simulink model "Multi_Robot_MPC_Adaptive"  (R2018a)
settings: Solver=VariableStepAuto  StartTime=0.0  StopTime=inf  FixedStep=sampleTime  RelTol=1e-3
PreLoadFcn:
  | % Simulation parameters
  | load exampleMap
  | sampleTime = 0.05;
  | 
  | % Robot parameters
  | wheelRadius = 0.025;
  | robotRadius = 0.35;
  | 
  | % Lidar parameters
  | sensorOffset = [0,0];
  | scanAngles = linspace(-pi/2,pi/2,9)';
  | maxRange = 5;
undefined symbols (not defined in the file): Ad, Bd, Beta, C1, C2, cBW, d, dw, Kb, Kg, Kt, L, La, magnitude, mc, R, Ra, Waypoint
libraries: mobileRoboticsLib x7, cstblocks x1, dspsrcs4 x1
settings Model: EnablePacing=on  Creator=scastro  LastModifiedBy=shravan

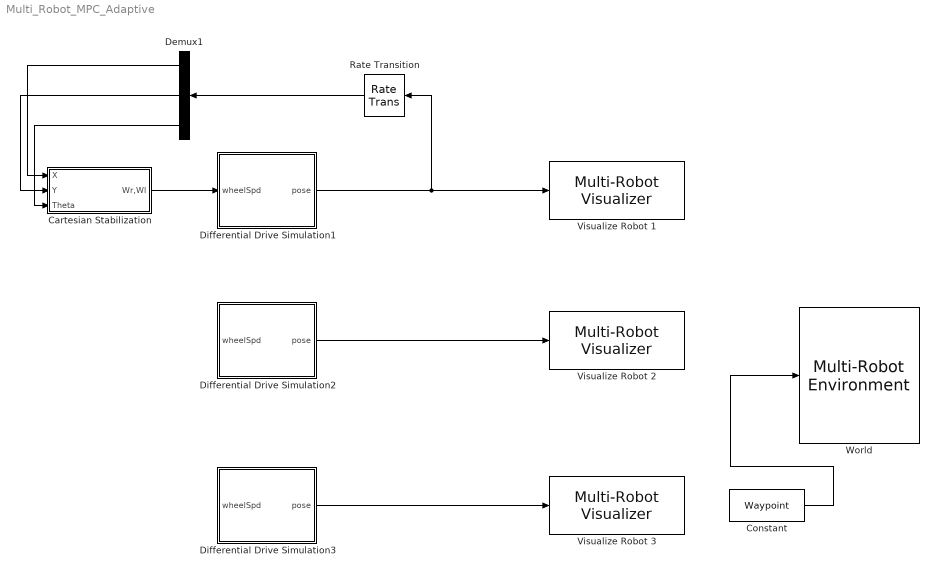
== system Multi_Robot_MPC_Adaptive ==
  Cartesian Stabilization : Subsystem
  Constant : Constant  Value=Waypoint  SampleTime=sampleTime
  Demux1 : Demux  Outputs=3
  Differential Drive Simulation1 : Subsystem  AncestorBlock=mobileRoboticsLib/Kinematic Models/Differential Drive/Differential Drive Simulation  OverrideUsingVariant=mode==2  mask(Differential Drive Simulation){wheelRadius=R, wheelBase=L, initX=C1, initY=C2, initAngle=0, Ts=0}
      mask prompts: wheelRadius "Wheel Radius [m]"; wheelBase "Wheelbase [m]"; initX "Initial X Position [m]"; initY "Initial Y Position [m]"; initAngle "Initial Angle [rad]"; Ts "Sample Time"
      mask help:
      | Simulates the kinematics of a differential drive vehicle from a specified initial pose.
      |
      | Input: Left and right wheel speeds [wL; wR], in rad/s
      |
      | Output: Pose [x; y; theta], in m, m, and rad
      |
      | Set the Sample Time parameter to 0 for continuous-time simulation, or a positive number for discrete-time simulation.
      mask Help: web('matlab:edit mrsDocDifferentialDrive')
      mask Callback Ts:
      | Ts = evalin('base',get_param(gcb,'Ts'));
      | blk = [gcb '/Generic Robot Simulation/Velocity Integrator'];
      | if Ts > 0
      |     set_param(blk,'OverrideUsingVariant','mode==2');
      | else
      |     set_param(blk,'OverrideUsingVariant','mode==1');
      | end
  Differential Drive Simulation2 : Subsystem  AncestorBlock=mobileRoboticsLib/Kinematic Models/Differential Drive/Differential Drive Simulation  OverrideUsingVariant=mode==2  mask(Differential Drive Simulation){wheelRadius=R, wheelBase=L, initX=C1, initY=C2+1, initAngle=0, Ts=0}
      mask prompts: wheelRadius "Wheel Radius [m]"; wheelBase "Wheelbase [m]"; initX "Initial X Position [m]"; initY "Initial Y Position [m]"; initAngle "Initial Angle [rad]"; Ts "Sample Time"
      mask help:
      | Simulates the kinematics of a differential drive vehicle from a specified initial pose.
      |
      | Input: Left and right wheel speeds [wL; wR], in rad/s
      |
      | Output: Pose [x; y; theta], in m, m, and rad
      |
      | Set the Sample Time parameter to 0 for continuous-time simulation, or a positive number for discrete-time simulation.
      mask Help: web('matlab:edit mrsDocDifferentialDrive')
      mask Callback Ts:
      | Ts = evalin('base',get_param(gcb,'Ts'));
      | blk = [gcb '/Generic Robot Simulation/Velocity Integrator'];
      | if Ts > 0
      |     set_param(blk,'OverrideUsingVariant','mode==2');
      | else
      |     set_param(blk,'OverrideUsingVariant','mode==1');
      | end
  Differential Drive Simulation3 : Subsystem  AncestorBlock=mobileRoboticsLib/Kinematic Models/Differential Drive/Differential Drive Simulation  OverrideUsingVariant=mode==2  mask(Differential Drive Simulation){wheelRadius=R, wheelBase=L, initX=C1, initY=C2-1, initAngle=0, Ts=0}
      mask prompts: wheelRadius "Wheel Radius [m]"; wheelBase "Wheelbase [m]"; initX "Initial X Position [m]"; initY "Initial Y Position [m]"; initAngle "Initial Angle [rad]"; Ts "Sample Time"
      mask help:
      | Simulates the kinematics of a differential drive vehicle from a specified initial pose.
      |
      | Input: Left and right wheel speeds [wL; wR], in rad/s
      |
      | Output: Pose [x; y; theta], in m, m, and rad
      |
      | Set the Sample Time parameter to 0 for continuous-time simulation, or a positive number for discrete-time simulation.
      mask Help: web('matlab:edit mrsDocDifferentialDrive')
      mask Callback Ts:
      | Ts = evalin('base',get_param(gcb,'Ts'));
      | blk = [gcb '/Generic Robot Simulation/Velocity Integrator'];
      | if Ts > 0
      |     set_param(blk,'OverrideUsingVariant','mode==2');
      | else
      |     set_param(blk,'OverrideUsingVariant','mode==1');
      | end
  Rate Transition : RateTransition  OutPortSampleTime=0.01
  Visualize Robot 1 : mobileRoboticsLib/Environments/Multi-Robot Visualizer  idx=1  radius=0.8  robotColor=[0 0 1]  showTraj=on  hasLidar=off  sensorOffset=[0 0]  scanAngles=[-pi/4,0,pi/4]  hasObjDetector=off  objDetectorOffset=[0;0]  objDetectorAngle=0  objDetectorFOV=pi/2  objDetectorMaxRange=5
      settings: SourceProductName=Mobile Robotics Simulation Toolbox
  Visualize Robot 2 : mobileRoboticsLib/Environments/Multi-Robot Visualizer  idx=2  radius=0.8  robotColor=[0 1 0]  showTraj=on  hasLidar=off  sensorOffset=[0 0]  scanAngles=[-pi/4,0,pi/4]  hasObjDetector=off  objDetectorOffset=[0;0]  objDetectorAngle=0  objDetectorFOV=pi/2  objDetectorMaxRange=5
      settings: SourceProductName=Mobile Robotics Simulation Toolbox
  Visualize Robot 3 : mobileRoboticsLib/Environments/Multi-Robot Visualizer  idx=3  radius=0.8  robotColor=[1 0 1]  showTraj=on  hasLidar=off  sensorOffset=[0 0]  scanAngles=[-pi/4,0,pi/4]  hasObjDetector=off  objDetectorOffset=[0;0]  objDetectorAngle=0  objDetectorFOV=pi/2  objDetectorMaxRange=5
      settings: SourceProductName=Mobile Robotics Simulation Toolbox
  World : mobileRoboticsLib/Environments/Multi-Robot Environment  numRobots=3  showWaypoints=on  showObjects=off  objectColors=[1 0 0;0 1 0;0 0 1]  objectMarkers='s'  showRobotIds=on  plotSensorLines=off
      settings: SourceProductName=Mobile Robotics Simulation Toolbox
  wires:
  Differential Drive Simulation1/1(pose) -> Rate Transition/1, Visualize Robot 1/1
  Cartesian Stabilization/1(Wr,Wl) -> Differential Drive Simulation1/1(wheelSpd)
  Rate Transition/1 -> Demux1/1
  Demux1/1 -> Cartesian Stabilization/1(X)
  Demux1/2 -> Cartesian Stabilization/2(Y)
  Demux1/3 -> Cartesian Stabilization/3(Theta)
  Differential Drive Simulation2/1(pose) -> Visualize Robot 2/1
  Differential Drive Simulation3/1(pose) -> Visualize Robot 3/1
  Constant/1 -> World/1

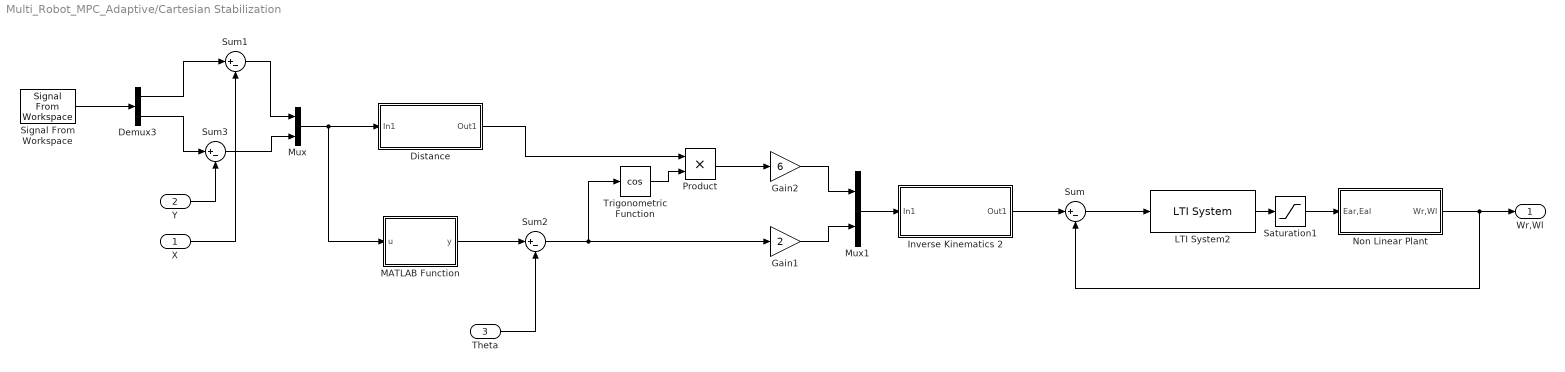
== system Multi_Robot_MPC_Adaptive/Cartesian Stabilization ==
  X : Inport
  Y : Inport  Port=2
  Theta : Inport  Port=3
  Demux3 : Demux  Outputs=2
  "Distance " : Subsystem
  Gain1 : Gain  Gain=2
  Gain2 : Gain  Gain=6
  Inverse Kinematics 2 : Subsystem
  LTI System2 : cstblocks/LTI System  sys=Controller  IC=[]
  MATLAB Function : MATLAB Function  TreatAsAtomicUnit=on
  Mux : Mux  Inputs=2
  Mux1 : Mux  Inputs=2
  "Non Linear Plant " : Subsystem
  Product : Product
  Saturation1 : Saturate  UpperLimit=30  LowerLimit=-30
  Signal From Workspace : dspsrcs4/Signal From Workspace  X=Cartesian  Ts=cBW  nsamps=1  OutputAfterFinalValue=Holding final value  ignoreOrWarnInputAndFrameLengths=off  OutputFrames=off
  Sum{,1..3} (4 alike) : Sum  Inputs=|+-
  Trigonometric Function : Trigonometry  Operator=cos
  Wr,Wl : Outport
  wires:
  "Distance "/1(Out1) -> Product/1
  Y/1 -> Sum3/2
  Demux3/1 -> Sum1/1
  Saturation1/1 -> "Non Linear Plant "/1(Ear,Eal)
  Gain2/1 -> Mux1/1
  Mux1/1 -> Inverse Kinematics 2/1(In1)
  Sum1/1 -> Mux/1
  Demux3/2 -> Sum3/1
  LTI System2/1 -> Saturation1/1
  Inverse Kinematics 2/1(Out1) -> Sum/1
  Signal From Workspace/1 -> Demux3/1
  Gain1/1 -> Mux1/2
  Sum3/1 -> Mux/2
  Theta/1 -> Sum2/2
  Sum/1 -> LTI System2/1
  "Non Linear Plant "/1(Wr,Wl) -> Wr,Wl/1, Sum/2
  Trigonometric Function/1 -> Product/2
  MATLAB Function/1(y) -> Sum2/1
  X/1 -> Sum1/2
  Product/1 -> Gain2/1
  Sum2/1 -> Gain1/1, Trigonometric Function/1
  Mux/1 -> MATLAB Function/1(u), "Distance "/1(In1)

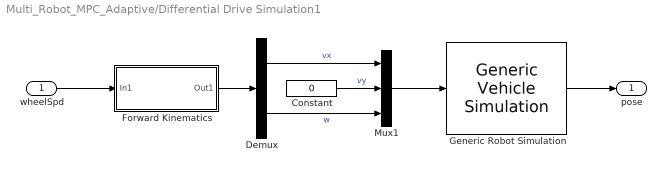
== system Multi_Robot_MPC_Adaptive/Differential Drive Simulation1 ==
  wheelSpd : Inport
  Constant : Constant  Value=0
  Demux : Demux  Outputs=2
  "Forward Kinematics " : Subsystem
  Generic Robot Simulation : mobileRoboticsLib/Utilities/Generic Vehicle Simulation  initX=initX  initY=initY  initAngle=initAngle  Ts=Ts
      link override Velocity Integrator: OverrideUsingVariant=mode==1
      settings: SourceProductName=Mobile Robotics Simulation Toolbox
  Mux1 : Mux  Inputs=3
  pose : Outport
  wires:
  Mux1/1 -> Generic Robot Simulation/1
  Demux/1 -> Mux1/1  "vx"
  Demux/2 -> Mux1/3  "w"
  Constant/1 -> Mux1/2  "vy"
  wheelSpd/1 -> "Forward Kinematics "/1(In1)
  "Forward Kinematics "/1(Out1) -> Demux/1
  Generic Robot Simulation/1 -> pose/1

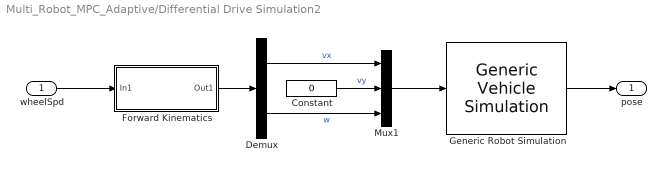
== system Multi_Robot_MPC_Adaptive/Differential Drive Simulation2 ==
  wheelSpd : Inport
  Constant : Constant  Value=0
  Demux : Demux  Outputs=2
  "Forward Kinematics " : Subsystem
  Generic Robot Simulation : mobileRoboticsLib/Utilities/Generic Vehicle Simulation  initX=initX  initY=initY  initAngle=initAngle  Ts=Ts
      link override Velocity Integrator: OverrideUsingVariant=mode==1
      settings: SourceProductName=Mobile Robotics Simulation Toolbox
  Mux1 : Mux  Inputs=3
  pose : Outport
  wires:
  Mux1/1 -> Generic Robot Simulation/1
  Demux/1 -> Mux1/1  "vx"
  Demux/2 -> Mux1/3  "w"
  Constant/1 -> Mux1/2  "vy"
  wheelSpd/1 -> "Forward Kinematics "/1(In1)
  "Forward Kinematics "/1(Out1) -> Demux/1
  Generic Robot Simulation/1 -> pose/1

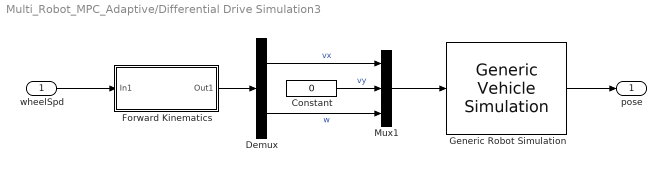
== system Multi_Robot_MPC_Adaptive/Differential Drive Simulation3 ==
  wheelSpd : Inport
  Constant : Constant  Value=0
  Demux : Demux  Outputs=2
  "Forward Kinematics " : Subsystem
  Generic Robot Simulation : mobileRoboticsLib/Utilities/Generic Vehicle Simulation  initX=initX  initY=initY  initAngle=initAngle  Ts=Ts
      link override Velocity Integrator: OverrideUsingVariant=mode==1
      settings: SourceProductName=Mobile Robotics Simulation Toolbox
  Mux1 : Mux  Inputs=3
  pose : Outport
  wires:
  Mux1/1 -> Generic Robot Simulation/1
  Demux/1 -> Mux1/1  "vx"
  Demux/2 -> Mux1/3  "w"
  Constant/1 -> Mux1/2  "vy"
  wheelSpd/1 -> "Forward Kinematics "/1(In1)
  "Forward Kinematics "/1(Out1) -> Demux/1
  Generic Robot Simulation/1 -> pose/1

== system Multi_Robot_MPC_Adaptive/Cartesian Stabilization/Distance  ==
  In1 : Inport
  Add2 : Sum
  Demux : Demux  Outputs=2
  Math Function : Math  Operator=magnitude^2  SaturateOnIntegerOverflow=on
  Math Function1 : Math  Operator=magnitude^2  SaturateOnIntegerOverflow=on
  Sqrt : Sqrt  SaturateOnIntegerOverflow=on
  Out1 : Outport
  wires:
  In1/1 -> Demux/1
  Demux/1 -> Math Function/1
  Demux/2 -> Math Function1/1
  Math Function/1 -> Add2/1
  Math Function1/1 -> Add2/2
  Add2/1 -> Sqrt/1
  Sqrt/1 -> Out1/1

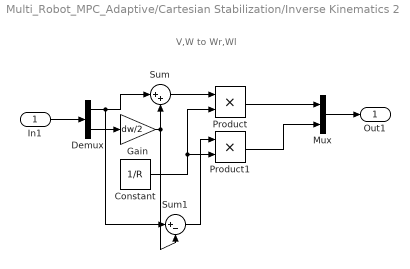
== system Multi_Robot_MPC_Adaptive/Cartesian Stabilization/Inverse Kinematics 2 ==
  note: V,W to Wr,Wl
  In1 : Inport
  Constant : Constant  Value=1/R
  Demux : Demux  Outputs=2
  Gain : Gain  Gain=dw/2
  Mux : Mux  Inputs=2
  Product : Product
  Product1 : Product
  Sum : Sum  Inputs=|++
  Sum1 : Sum  Inputs=|+-
  Out1 : Outport
  wires:
  Mux/1 -> Out1/1
  In1/1 -> Demux/1
  Demux/2 -> Gain/1
  Demux/1 -> Sum1/1, Sum/1
  Gain/1 -> Sum1/2, Sum/2
  Sum/1 -> Product/1
  Constant/1 -> Product1/2, Product/2
  Sum1/1 -> Product1/1
  Product/1 -> Mux/1
  Product1/1 -> Mux/2

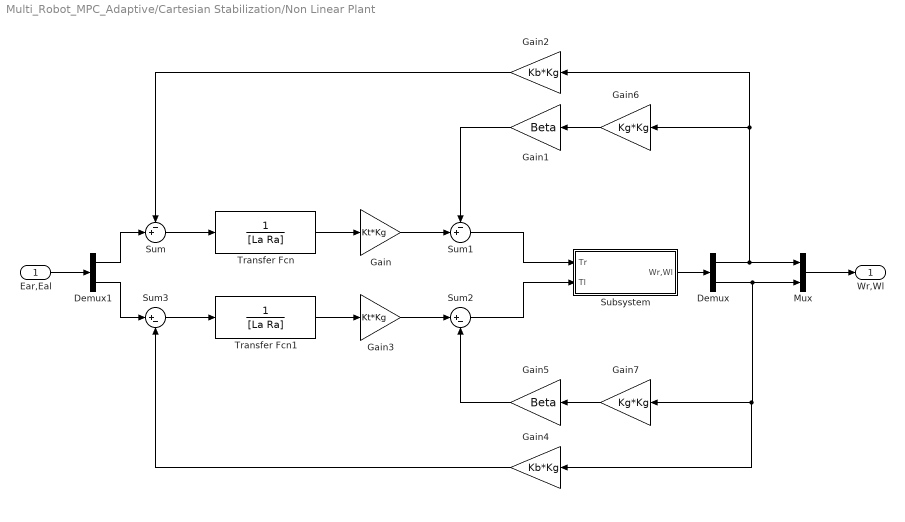
== system Multi_Robot_MPC_Adaptive/Cartesian Stabilization/Non Linear Plant  ==
  Ear,Eal : Inport
  Demux : Demux  Outputs=2
  Demux1 : Demux  Outputs=2
  Gain : Gain  Gain=Kt*Kg
  Gain1 : Gain  Gain=Beta
  Gain2 : Gain  Gain=Kb*Kg
  Gain3 : Gain  Gain=Kt*Kg
  Gain4 : Gain  Gain=Kb*Kg
  Gain5 : Gain  Gain=Beta
  Gain6 : Gain  Gain=Kg*Kg
  Gain7 : Gain  Gain=Kg*Kg
  Mux : Mux  Inputs=2
  Subsystem : Subsystem
  Sum : Sum  Inputs=-+|
  Sum1 : Sum  Inputs=-+|
  Sum2 : Sum  Inputs=|+-
  Sum3 : Sum  Inputs=|+-
  Transfer Fcn : TransferFcn  Denominator=[La Ra]
  Transfer Fcn1 : TransferFcn  Denominator=[La Ra]
  Wr,Wl : Outport
  wires:
  Gain5/1 -> Sum2/2
  Gain4/1 -> Sum3/2
  Sum/1 -> Transfer Fcn/1
  Demux1/2 -> Sum3/1
  Gain1/1 -> Sum1/1
  Demux/1 -> Mux/1, Gain2/1, Gain6/1
  Subsystem/1(Wr,Wl) -> Demux/1
  Demux1/1 -> Sum/2
  Sum3/1 -> Transfer Fcn1/1
  Mux/1 -> Wr,Wl/1
  Gain2/1 -> Sum/1
  Gain/1 -> Sum1/2
  Ear,Eal/1 -> Demux1/1
  Sum1/1 -> Subsystem/1(Tr)
  Transfer Fcn/1 -> Gain/1
  Transfer Fcn1/1 -> Gain3/1
  Gain3/1 -> Sum2/1
  Demux/2 -> Mux/2, Gain4/1, Gain7/1
  Sum2/1 -> Subsystem/2(Tl)
  Gain6/1 -> Gain1/1
  Gain7/1 -> Gain5/1

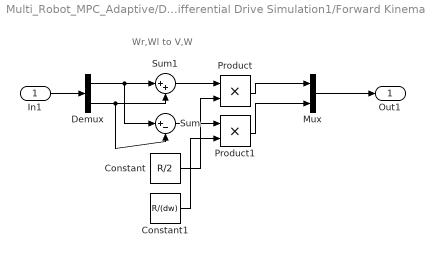
== system Multi_Robot_MPC_Adaptive/Differential Drive Simulation1/Forward Kinematics  ==
  note: Wr,Wl to V,W
  In1 : Inport
  Constant : Constant  Value=R/2
  Constant1 : Constant  Value=R/(dw)
  Demux : Demux  Outputs=2
  Mux : Mux  Inputs=2
  Product : Product
  Product1 : Product
  Sum : Sum  Inputs=|+-
  Sum1 : Sum  Inputs=|++
  Out1 : Outport
  wires:
  Product1/1 -> Mux/2
  Sum1/1 -> Product/1
  Constant/1 -> Product/2
  Constant1/1 -> Product1/2
  Product/1 -> Mux/1
  Mux/1 -> Out1/1
  Demux/2 -> Sum1/2, Sum/2
  Demux/1 -> Sum1/1, Sum/1
  Sum/1 -> Product1/1
  In1/1 -> Demux/1

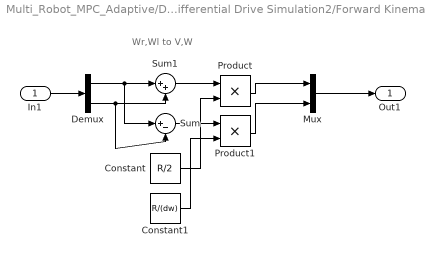
== system Multi_Robot_MPC_Adaptive/Differential Drive Simulation2/Forward Kinematics  ==
  note: Wr,Wl to V,W
  In1 : Inport
  Constant : Constant  Value=R/2
  Constant1 : Constant  Value=R/(dw)
  Demux : Demux  Outputs=2
  Mux : Mux  Inputs=2
  Product : Product
  Product1 : Product
  Sum : Sum  Inputs=|+-
  Sum1 : Sum  Inputs=|++
  Out1 : Outport
  wires:
  Product1/1 -> Mux/2
  Sum1/1 -> Product/1
  Constant/1 -> Product/2
  Constant1/1 -> Product1/2
  Product/1 -> Mux/1
  Mux/1 -> Out1/1
  Demux/2 -> Sum1/2, Sum/2
  Demux/1 -> Sum1/1, Sum/1
  Sum/1 -> Product1/1
  In1/1 -> Demux/1

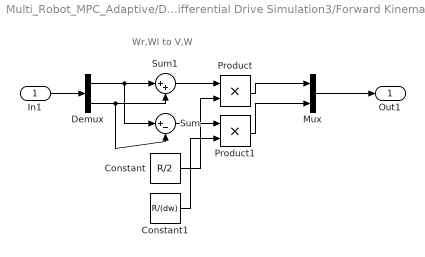
== system Multi_Robot_MPC_Adaptive/Differential Drive Simulation3/Forward Kinematics  ==
  note: Wr,Wl to V,W
  In1 : Inport
  Constant : Constant  Value=R/2
  Constant1 : Constant  Value=R/(dw)
  Demux : Demux  Outputs=2
  Mux : Mux  Inputs=2
  Product : Product
  Product1 : Product
  Sum : Sum  Inputs=|+-
  Sum1 : Sum  Inputs=|++
  Out1 : Outport
  wires:
  Product1/1 -> Mux/2
  Sum1/1 -> Product/1
  Constant/1 -> Product/2
  Constant1/1 -> Product1/2
  Product/1 -> Mux/1
  Mux/1 -> Out1/1
  Demux/2 -> Sum1/2, Sum/2
  Demux/1 -> Sum1/1, Sum/1
  Sum/1 -> Product1/1
  In1/1 -> Demux/1

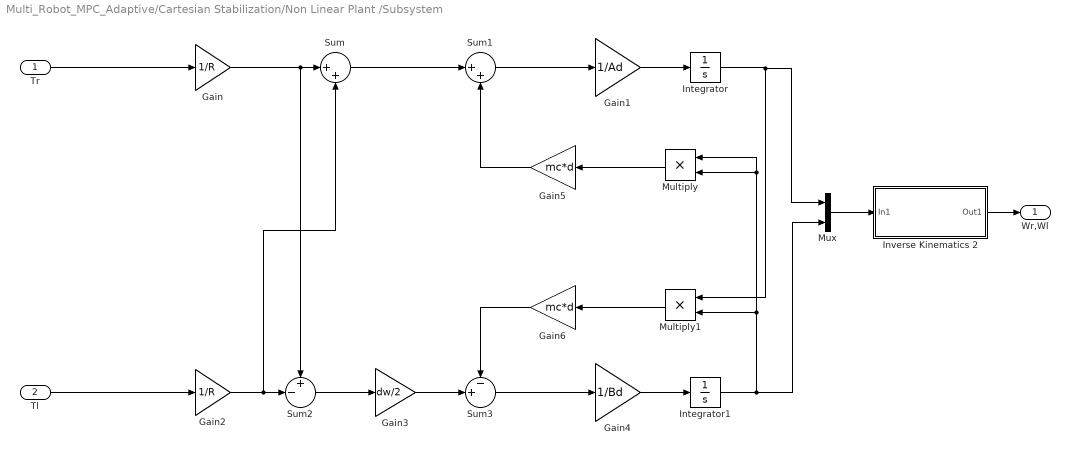
== system Multi_Robot_MPC_Adaptive/Cartesian Stabilization/Non Linear Plant /Subsystem ==
  Tr : Inport
  Tl : Inport  Port=2
  Gain : Gain  Gain=1/R
  Gain1 : Gain  Gain=1/Ad
  Gain2 : Gain  Gain=1/R
  Gain3 : Gain  Gain=dw/2
  Gain4 : Gain  Gain=1/Bd
  Gain5 : Gain  Gain=mc*d
  Gain6 : Gain  Gain=mc*d
  Integrator : Integrator
  Integrator1 : Integrator
  Inverse Kinematics 2 : Subsystem
  Multiply : Product
  Multiply1 : Product
  Mux : Mux  Inputs=2
  Sum : Sum  Inputs=|++
  Sum1 : Sum  Inputs=|++
  Sum2 : Sum  Inputs=+-|
  Sum3 : Sum  Inputs=-+|
  Wr,Wl : Outport
  wires:
  Sum1/1 -> Gain1/1
  Multiply1/1 -> Gain6/1
  Sum3/1 -> Gain4/1
  Gain/1 -> Sum/1, Sum2/1
  Integrator/1 -> Mux/1, Multiply1/1
  Mux/1 -> Inverse Kinematics 2/1(In1)
  Gain4/1 -> Integrator1/1
  Inverse Kinematics 2/1(Out1) -> Wr,Wl/1
  Sum/1 -> Sum1/1
  Gain5/1 -> Sum1/2
  Tr/1 -> Gain/1
  Integrator1/1 -> Multiply1/2, Multiply/2, Multiply/1, Mux/2
  Multiply/1 -> Gain5/1
  Gain3/1 -> Sum3/2
  Sum2/1 -> Gain3/1
  Gain2/1 -> Sum/2, Sum2/2
  Gain6/1 -> Sum3/1
  Tl/1 -> Gain2/1
  Gain1/1 -> Integrator/1

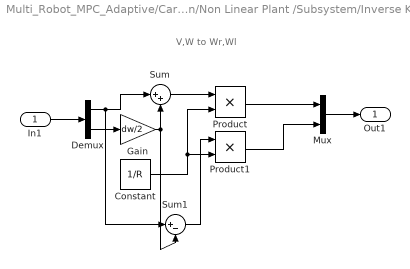
== system Multi_Robot_MPC_Adaptive/Cartesian Stabilization/Non Linear Plant /Subsystem/Inverse Kinematics 2 ==
  note: V,W to Wr,Wl
  In1 : Inport
  Constant : Constant  Value=1/R
  Demux : Demux  Outputs=2
  Gain : Gain  Gain=dw/2
  Mux : Mux  Inputs=2
  Product : Product
  Product1 : Product
  Sum : Sum  Inputs=|++
  Sum1 : Sum  Inputs=|+-
  Out1 : Outport
  wires:
  Mux/1 -> Out1/1
  In1/1 -> Demux/1
  Demux/2 -> Gain/1
  Demux/1 -> Sum1/1, Sum/1
  Gain/1 -> Sum1/2, Sum/2
  Sum/1 -> Product/1
  Constant/1 -> Product1/2, Product/2
  Sum1/1 -> Product1/1
  Product/1 -> Mux/1
  Product1/1 -> Mux/2

== matlab function Multi_Robot_MPC_Adaptive/Cartesian Stabilization/MATLAB Function ==
  data: u input size=2,1; y output size=1,1
function y = fcn(u)
persistent xo yo theta;
if isempty(xo)||isempty(yo)||isempty(theta)
    xo = 1; yo = 0; theta = 0;
end
xp = u(1,1); yp = u(2,1);

% calculate the value of theta
a1 = sqrt(xp^2 + yp^2);
b1 = sqrt(xo^2 + yo^2);
c1 = sqrt((xp - xo)^2 + (yp - yo)^2);
if (a1 ~= 0)&&(b1 ~= 0)  
    dtheta = acos(max(min((a1^2 + b1^2 - c1^2)/(2*a1*b1),1),-1));
else
    dtheta = 0;
end
% calculate the direction of rotation
sign = 1;
if dtheta ~= 0
    sign = (-yo/xo)*xp + yp;
    if sign ~= 0
        if (xo > 0)&&(yo > 0)
                sign = sign/abs(sign);
        elseif (xo < 0)&&(yo < 0)
                sign = -sign/abs(sign);
        elseif (xo > 0)&&(yo < 0)
                sign = sign/abs(sign);
        elseif (xo < 0)&&(yo > 0)
                 sign = -sign/abs(sign);
        elseif (xo == 0)&&(yo >= 0)
            if xp ~= 0
                sign = -xp/abs(xp);
            else
                sign = 0;
            end
        elseif (xo == 0)&&(yo <= 0)
            if xp ~= 0
                sign = xp/abs(xp);
            else
                sign = 0;
            end
        elseif (xo >= 0)&&(yo == 0)
            if yp ~= 0
                sign = yp/abs(yp);
            else
                sign = 0;
            end
        elseif ((xo <= 0)&&(yo == 0))
            if yp ~= 0
                sign = -yp/abs(yp);
            else
                sign = 0;
            end
        end
    end
end

xo = xp; yo = yp; 
theta = theta + dtheta*sign;
y = theta;
